simulink model "Proj_Model"  (R2015a)
settings: Solver=ode45  StartTime=0.0  StopTime=100.0  RelTol=1e-3
values from neighbouring files (symbols this model uses):
  d1 = 0.5    [mdl_data.m]    (also in proj_model.m = 0)
  d2 = 0.5    [mdl_data.m]    (also in proj_model.m = 0)
  d3 = 0.5    [mdl_data.m]    (also in proj_model.m = 0)
  d4 = 0.8    [mdl_data.m]    (also in proj_model.m = 0)
  d5 = 0.8    [mdl_data.m]    (also in proj_model.m = 0)
  d6 = 0.8    [mdl_data.m]    (also in proj_model.m = 0)
  del10 = 0.1    [mdl_data.m]    (also in proj_model.m)
  del20 = 0.11    [mdl_data.m]    (also in proj_model.m)
  del30 = 0.105    [mdl_data.m]    (also in proj_model.m)
  del40 = 0.21    [mdl_data.m]    (also in proj_model.m)
  del50 = 0.205    [mdl_data.m]    (also in proj_model.m)
  del60 = 0.211    [mdl_data.m]    (also in proj_model.m)
  K = lqr(A,B,Q,R,N)    [decoupled_des2.m]    (also in decoupled_model.m; proj_model.m = dlqr(sys_d.a,sys_d.b,Q,R))
  K12 = E1*E2/x12    (= 100)    [mdl_data.m]
  K13 = E1*E3/x31    (= 100)    [mdl_data.m]
  K23 = E3*E2/x23    (= 100)    [mdl_data.m]
  K26 = E6*E2/x26    (= 20)    [mdl_data.m]
  K31 = K13    (= 100)    [mdl_data.m]
  K32 = K23    (= 100)    [mdl_data.m]
  K46 = E4*E6/x64    (= 20)    [mdl_data.m]
  K54 = K45    (= 20)    [mdl_data.m]
  K56 = E5*E6/x56    (= 20)    [mdl_data.m]
  K62 = K26    (= 20)    [mdl_data.m]
  K64 = K46    (= 20)    [mdl_data.m]
  K65 = K56    (= 20)    [mdl_data.m]
  M1 = 1    [decoupled_des2.m]    (also in decoupled_model.m; mdl_data.m; proj_model.m)
  M2 = 1    [decoupled_des2.m]    (also in decoupled_model.m; mdl_data.m; proj_model.m)
  M3 = 1    [decoupled_des2.m]    (also in decoupled_model.m; mdl_data.m; proj_model.m)
  M4 = 2    [decoupled_des2.m]    (also in decoupled_model.m; mdl_data.m; proj_model.m)
  M5 = 2    [decoupled_des2.m]    (also in decoupled_model.m; mdl_data.m; proj_model.m)
  M6 = 2    [decoupled_des2.m]    (also in decoupled_model.m; mdl_data.m; proj_model.m)
settings Model: CovSFcnEnable=off  Creator=nchocka  LastModifiedBy=nachi
settings DebuggingCC: UnderspecifiedInitializationDetection=Classic  MergeDetectMultiDrivingBlocksExec=none  StateNameClashWarn=warning

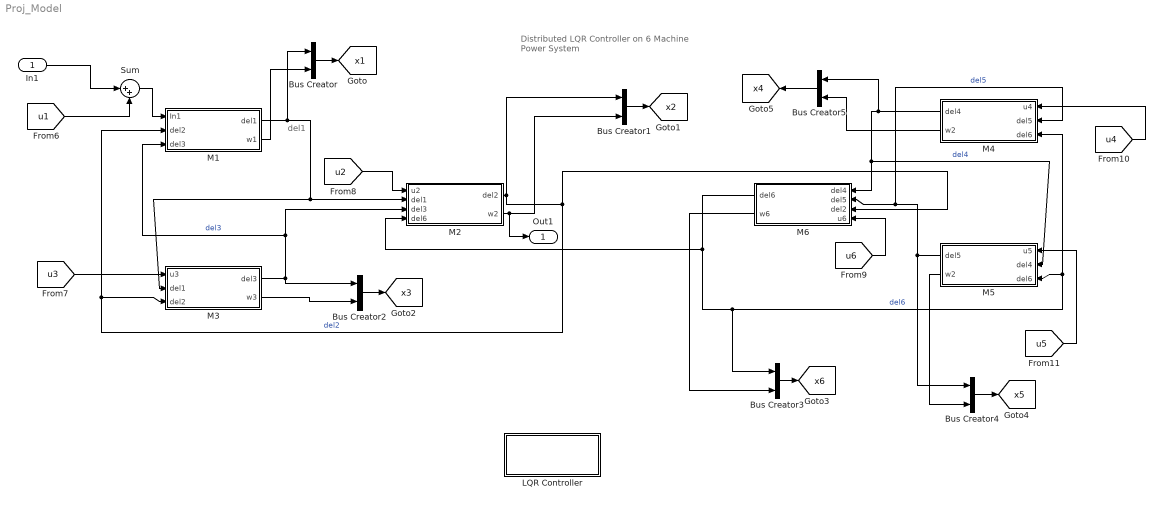
== system Proj_Model ==
  note: del1
  note: Distributed LQR Controller on 6 Machine Power System
  In1 : Inport
  Bus Creator{,1..5} (6 alike) : BusCreator  Inputs=2
  LQR Controller : Subsystem
  M1 : Subsystem
  M2 : Subsystem
  M3 : Subsystem
  M4 : Subsystem
  M5 : Subsystem
  M6 : Subsystem
  Sum : Sum  Inputs=|++
  Out1 : Outport
  tag scope: x1=global, x2=global, x3=global, x4=global, x5=global, x6=global
  wires:
  M1/1(del1) -> Bus Creator/1, M2/2(del1), M3/2(del1)
  M3/1(del3) -> M2/3(del3), M1/3(del3), Bus Creator2/1  "del3"
  M6/1(del6) -> Bus Creator3/1, M4/3(del6), M5/3(del6), M2/4(del6)  "del6"
  M2/1(del2) -> M1/2(del2), M3/3(del2), M6/3(del2), Bus Creator1/1  "del2"
  M4/1(del4) -> Bus Creator5/1, M5/2(del4), M6/1(del4)  "del4"
  M5/1(del5) -> Bus Creator4/1, M4/2(del5), M6/2(del5)  "del5"
  [u1] -> Sum/2
  [u6] -> M6/4(u6)
  M3/2(w3) -> Bus Creator2/2
  M5/2(w2) -> Bus Creator4/2
  M6/2(w6) -> Bus Creator3/2
  M4/2(w2) -> Bus Creator5/2
  M1/2(w1) -> Bus Creator/2
  Bus Creator/1 -> [x1]
  Bus Creator1/1 -> [x2]
  Bus Creator2/1 -> [x3]
  Bus Creator3/1 -> [x6]
  Bus Creator4/1 -> [x5]
  Bus Creator5/1 -> [x4]
  [u3] -> M3/1(u3)
  [u2] -> M2/1(u2)
  [u4] -> M4/1("u4 ")
  [u5] -> M5/1("u5 ")
  Sum/1 -> M1/1(In1)
  In1/1 -> Sum/1
  M2/2(w2) -> Out1/1, Bus Creator1/2

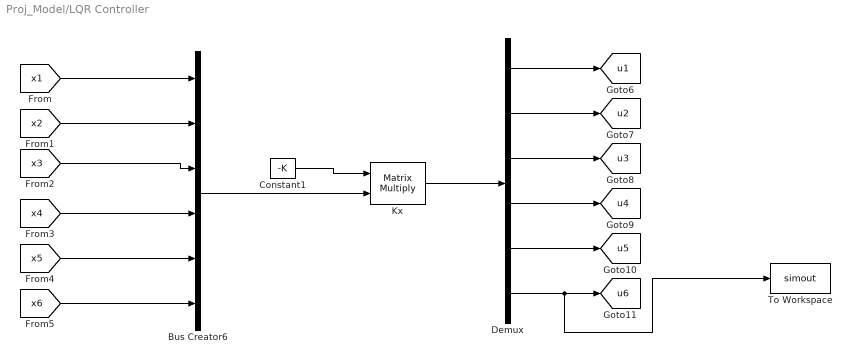
== system Proj_Model/LQR Controller ==
  Bus Creator6 : BusCreator  Inputs=6
  Constant1 : Constant  Value=-K
  Demux : Demux  Outputs=6
  Kx : Product  Multiplication=Matrix(*)
  To Workspace : ToWorkspace  VariableName=simout  SaveFormat=Timeseries  SampleTime=-1
  tag scope: u1=global, u2=global, u3=global, u4=global, u5=global, u6=global
  wires:
  [x6] -> Bus Creator6/6
  [x5] -> Bus Creator6/5
  [x3] -> Bus Creator6/3
  [x4] -> Bus Creator6/4
  [x2] -> Bus Creator6/2
  [x1] -> Bus Creator6/1
  Bus Creator6/1 -> Kx/2
  Kx/1 -> Demux/1
  Constant1/1 -> Kx/1
  Demux/1 -> [u1]
  Demux/2 -> [u2]
  Demux/3 -> [u3]
  Demux/4 -> [u4]
  Demux/5 -> [u5]
  Demux/6 -> To Workspace/1, [u6]

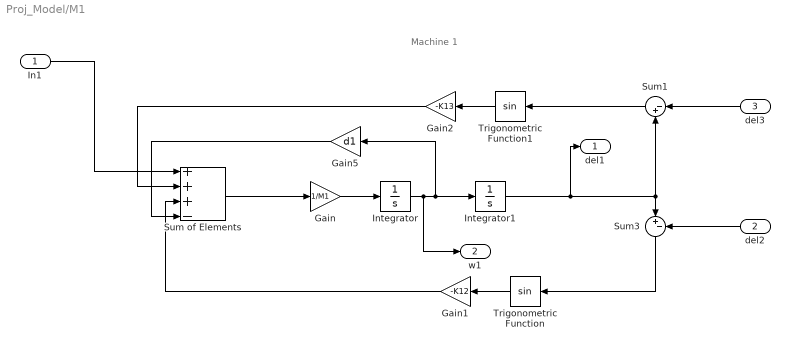
== system Proj_Model/M1 ==
  note: Machine 1
  In1 : Inport
  del2 : Inport  Port=2
  del3 : Inport  Port=3
  Gain : Gain  Gain=1/M1
  Gain1 : Gain  Gain=-K12
  Gain2 : Gain  Gain=-K13
  Gain5 : Gain  Gain=d1
  Integrator : Integrator
  Integrator1 : Integrator  InitialCondition=del10
  Sum of Elements : Sum  Inputs=+++-
  Sum1 : Sum  Inputs=|-+
  Sum3 : Sum  Inputs=|+-
  Trigonometric Function : Trigonometry
  Trigonometric Function1 : Trigonometry
  del1 : Outport
  w1 : Outport  Port=2
  wires:
  Integrator/1 -> w1/1, Gain5/1, Integrator1/1
  Gain/1 -> Integrator/1
  Integrator1/1 -> del1/1, Sum3/1, Sum1/2
  Sum3/1 -> Trigonometric Function/1
  Sum of Elements/1 -> Gain/1
  Trigonometric Function/1 -> Gain1/1
  Gain1/1 -> Sum of Elements/3
  Gain5/1 -> Sum of Elements/4
  del2/1 -> Sum3/2
  del3/1 -> Sum1/1
  Trigonometric Function1/1 -> Gain2/1
  Sum1/1 -> Trigonometric Function1/1
  Gain2/1 -> Sum of Elements/2
  In1/1 -> Sum of Elements/1

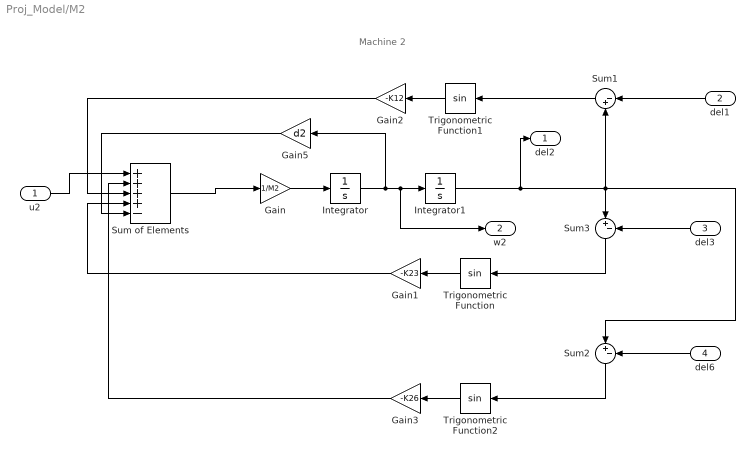
== system Proj_Model/M2 ==
  note: Machine 2
  u2 : Inport
  del1 : Inport  Port=2
  del3 : Inport  Port=3
  del6 : Inport  Port=4
  Gain : Gain  Gain=1/M2
  Gain1 : Gain  Gain=-K23
  Gain2 : Gain  Gain=-K12
  Gain3 : Gain  Gain=-K26
  Gain5 : Gain  Gain=d2
  Integrator : Integrator
  Integrator1 : Integrator  InitialCondition=del20
  Sum of Elements : Sum  Inputs=++++-
  Sum1 : Sum  Inputs=|-+
  Sum2 : Sum  Inputs=|+-
  Sum3 : Sum  Inputs=|+-
  Trigonometric Function : Trigonometry
  Trigonometric Function1 : Trigonometry
  Trigonometric Function2 : Trigonometry
  del2 : Outport
  w2 : Outport  Port=2
  wires:
  Integrator/1 -> Gain5/1, w2/1, Integrator1/1
  Gain/1 -> Integrator/1
  Sum3/1 -> Trigonometric Function/1
  Sum of Elements/1 -> Gain/1
  Trigonometric Function/1 -> Gain1/1
  Gain1/1 -> Sum of Elements/4
  Gain5/1 -> Sum of Elements/5
  del3/1 -> Sum3/2
  del1/1 -> Sum1/1
  Trigonometric Function1/1 -> Gain2/1
  Sum1/1 -> Trigonometric Function1/1
  Gain2/1 -> Sum of Elements/3
  Integrator1/1 -> del2/1, Sum2/1, Sum3/1, Sum1/2
  Sum2/1 -> Trigonometric Function2/1
  Trigonometric Function2/1 -> Gain3/1
  Gain3/1 -> Sum of Elements/2
  del6/1 -> Sum2/2
  u2/1 -> Sum of Elements/1

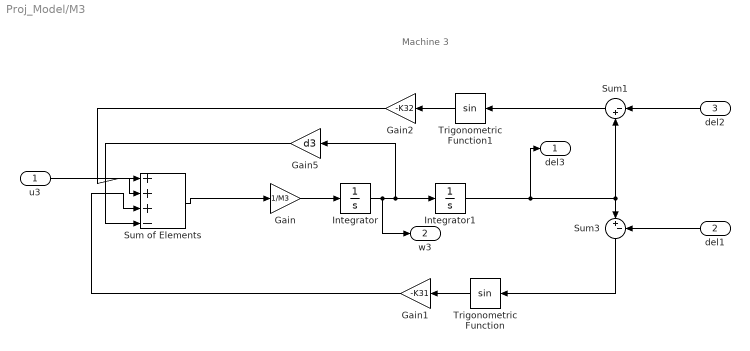
== system Proj_Model/M3 ==
  note: Machine 3
  u3 : Inport
  del1 : Inport  Port=2
  del2 : Inport  Port=3
  Gain : Gain  Gain=1/M3
  Gain1 : Gain  Gain=-K31
  Gain2 : Gain  Gain=-K32
  Gain5 : Gain  Gain=d3
  Integrator : Integrator
  Integrator1 : Integrator  InitialCondition=del30
  Sum of Elements : Sum  Inputs=+++-
  Sum1 : Sum  Inputs=|-+
  Sum3 : Sum  Inputs=|+-
  Trigonometric Function : Trigonometry
  Trigonometric Function1 : Trigonometry
  del3 : Outport
  w3 : Outport  Port=2
  wires:
  Gain2/1 -> Sum of Elements/2
  Sum1/1 -> Trigonometric Function1/1
  Trigonometric Function1/1 -> Gain2/1
  del2/1 -> Sum1/1
  del1/1 -> Sum3/2
  Gain5/1 -> Sum of Elements/4
  Gain1/1 -> Sum of Elements/3
  Trigonometric Function/1 -> Gain1/1
  Sum of Elements/1 -> Gain/1
  Sum3/1 -> Trigonometric Function/1
  Integrator1/1 -> Sum1/2, Sum3/1, del3/1
  Gain/1 -> Integrator/1
  Integrator/1 -> w3/1, Integrator1/1, Gain5/1
  u3/1 -> Sum of Elements/1

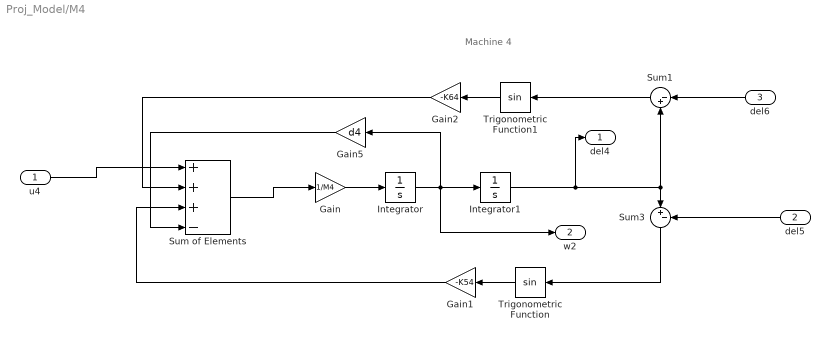
== system Proj_Model/M4 ==
  note: Machine 4
  "u4 " : Inport
  del5 : Inport  Port=2
  del6 : Inport  Port=3
  Gain : Gain  Gain=1/M4
  Gain1 : Gain  Gain=-K54
  Gain2 : Gain  Gain=-K64
  Gain5 : Gain  Gain=d4
  Integrator : Integrator
  Integrator1 : Integrator  InitialCondition=del40
  Sum of Elements : Sum  Inputs=+++-
  Sum1 : Sum  Inputs=|-+
  Sum3 : Sum  Inputs=|+-
  Trigonometric Function : Trigonometry
  Trigonometric Function1 : Trigonometry
  del4 : Outport
  w2 : Outport  Port=2
  wires:
  Integrator/1 -> w2/1, Gain5/1, Integrator1/1
  Gain/1 -> Integrator/1
  Integrator1/1 -> del4/1, Sum3/1, Sum1/2
  Sum3/1 -> Trigonometric Function/1
  Sum of Elements/1 -> Gain/1
  Trigonometric Function/1 -> Gain1/1
  Gain1/1 -> Sum of Elements/3
  Gain5/1 -> Sum of Elements/4
  del5/1 -> Sum3/2
  del6/1 -> Sum1/1
  Trigonometric Function1/1 -> Gain2/1
  Sum1/1 -> Trigonometric Function1/1
  Gain2/1 -> Sum of Elements/2
  "u4 "/1 -> Sum of Elements/1

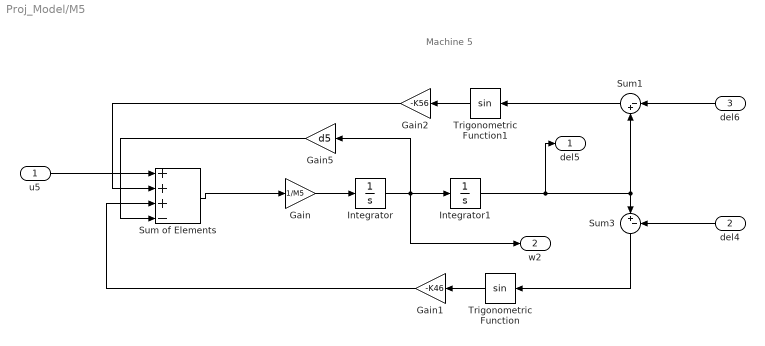
== system Proj_Model/M5 ==
  note: Machine 5
  "u5 " : Inport
  del4 : Inport  Port=2
  del6 : Inport  Port=3
  Gain : Gain  Gain=1/M5
  Gain1 : Gain  Gain=-K46
  Gain2 : Gain  Gain=-K56
  Gain5 : Gain  Gain=d5
  Integrator : Integrator
  Integrator1 : Integrator  InitialCondition=del50
  Sum of Elements : Sum  Inputs=+++-
  Sum1 : Sum  Inputs=|-+
  Sum3 : Sum  Inputs=|+-
  Trigonometric Function : Trigonometry
  Trigonometric Function1 : Trigonometry
  del5 : Outport
  w2 : Outport  Port=2
  wires:
  Gain2/1 -> Sum of Elements/2
  Sum1/1 -> Trigonometric Function1/1
  Trigonometric Function1/1 -> Gain2/1
  del6/1 -> Sum1/1
  del4/1 -> Sum3/2
  Gain5/1 -> Sum of Elements/4
  Gain1/1 -> Sum of Elements/3
  Trigonometric Function/1 -> Gain1/1
  Sum of Elements/1 -> Gain/1
  Sum3/1 -> Trigonometric Function/1
  Integrator1/1 -> Sum1/2, Sum3/1, del5/1
  Gain/1 -> Integrator/1
  Integrator/1 -> w2/1, Integrator1/1, Gain5/1
  "u5 "/1 -> Sum of Elements/1

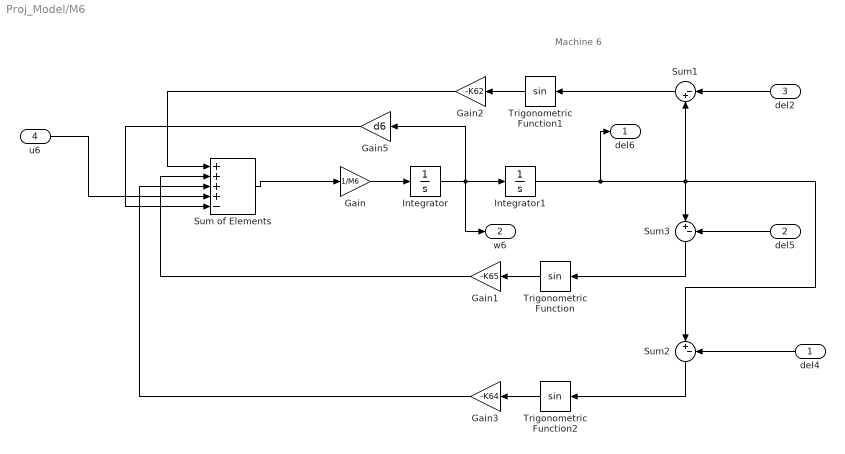
== system Proj_Model/M6 ==
  note: Machine 6
  del4 : Inport
  del5 : Inport  Port=2
  del2 : Inport  Port=3
  u6 : Inport  Port=4
  Gain : Gain  Gain=1/M6
  Gain1 : Gain  Gain=-K65
  Gain2 : Gain  Gain=-K62
  Gain3 : Gain  Gain=-K64
  Gain5 : Gain  Gain=d6
  Integrator : Integrator
  Integrator1 : Integrator  InitialCondition=del60
  Sum of Elements : Sum  Inputs=++++-
  Sum1 : Sum  Inputs=|-+
  Sum2 : Sum  Inputs=|+-
  Sum3 : Sum  Inputs=|+-
  Trigonometric Function : Trigonometry
  Trigonometric Function1 : Trigonometry
  Trigonometric Function2 : Trigonometry
  del6 : Outport
  w6 : Outport  Port=2
  wires:
  Gain2/1 -> Sum of Elements/1
  Sum1/1 -> Trigonometric Function1/1
  Trigonometric Function1/1 -> Gain2/1
  del2/1 -> Sum1/1
  del5/1 -> Sum3/2
  Gain1/1 -> Sum of Elements/2
  Trigonometric Function/1 -> Gain1/1
  Sum of Elements/1 -> Gain/1
  Sum3/1 -> Trigonometric Function/1
  Gain/1 -> Integrator/1
  Integrator/1 -> w6/1, Integrator1/1, Gain5/1
  del4/1 -> Sum2/2
  Gain3/1 -> Sum of Elements/3
  Trigonometric Function2/1 -> Gain3/1
  Sum2/1 -> Trigonometric Function2/1
  Integrator1/1 -> Sum2/1, Sum1/2, Sum3/1, del6/1
  Gain5/1 -> Sum of Elements/5
  u6/1 -> Sum of Elements/4
